simulink model "FanCtl_Spd"  (R2016b)
settings: configuration reference "CodeGenConfigSet" (kept outside this file)
values from neighbouring files (symbols this model uses):
  Fan_numFans_C = Calibration.Parameter    [init_FanCtl_Spd.m]    (also in init_FanCtl_Spd_SIL.m = Simulink.Parameter)
  Fan_rHys2Hi_C = Calibration.Parameter    [init_FanCtl_Spd.m]    (also in init_FanCtl_Spd_SIL.m = Simulink.Parameter)
  Fan_rHys2Lo_C = Calibration.Parameter    [init_FanCtl_Spd.m]    (also in init_FanCtl_Spd_SIL.m = Simulink.Parameter)
  Fan_rHysHi_C = Calibration.Parameter    [init_FanCtl_Spd.m]    (also in init_FanCtl_Spd_SIL.m = Simulink.Parameter)
  Fan_rHysLo_C = Calibration.Parameter    [init_FanCtl_Spd.m]    (also in init_FanCtl_Spd_SIL.m = Simulink.Parameter)
  FanCtl_facCorErr_C = Calibration.Parameter    [init_FanCtl_Spd.m]    (also in init_FanCtl_Spd_SIL.m = Simulink.Parameter)
  FanCtl_facCorSpd2_MAP = Calibration.Parameter    [init_FanCtl_Spd.m]    (also in init_FanCtl_Spd_SIL.m = Simulink.Parameter)
  FanCtl_facCorSpd2_MAPX = Calibration.Parameter    [init_FanCtl_Spd.m]    (also in init_FanCtl_Spd_SIL.m = Simulink.Parameter)
  FanCtl_facCorSpd2_MAPY = Calibration.Parameter    [init_FanCtl_Spd.m]    (also in init_FanCtl_Spd_SIL.m = Simulink.Parameter)
  FanCtl_facCorSpd_MAP = Calibration.Parameter    [init_FanCtl_Spd.m]    (also in init_FanCtl_Spd_SIL.m = Simulink.Parameter)
  FanCtl_facCorSpd_MAPX = Calibration.Parameter    [init_FanCtl_Spd.m]    (also in init_FanCtl_Spd_SIL.m = Simulink.Parameter)
  FanCtl_facCorSpd_MAPY = Calibration.Parameter    [init_FanCtl_Spd.m]    (also in init_FanCtl_Spd_SIL.m = Simulink.Parameter)
  FanCtl_nSpd2Win1L_C = Calibration.Parameter    [init_FanCtl_Spd.m]    (also in init_FanCtl_Spd_SIL.m = Simulink.Parameter)
  FanCtl_nSpd2Win1R_C = Calibration.Parameter    [init_FanCtl_Spd.m]    (also in init_FanCtl_Spd_SIL.m = Simulink.Parameter)
  FanCtl_nSpd2Win2L_C = Calibration.Parameter    [init_FanCtl_Spd.m]    (also in init_FanCtl_Spd_SIL.m = Simulink.Parameter)
  FanCtl_nSpd2Win2R_C = Calibration.Parameter    [init_FanCtl_Spd.m]    (also in init_FanCtl_Spd_SIL.m = Simulink.Parameter)
  FanCtl_nSpd2Win3L_C = Calibration.Parameter    [init_FanCtl_Spd.m]    (also in init_FanCtl_Spd_SIL.m = Simulink.Parameter)
  FanCtl_nSpd2Win3R_C = Calibration.Parameter    [init_FanCtl_Spd.m]    (also in init_FanCtl_Spd_SIL.m = Simulink.Parameter)
  FanCtl_nSpdDes2_MAP = Calibration.Parameter    [init_FanCtl_Spd.m]    (also in init_FanCtl_Spd_SIL.m = Simulink.Parameter)
  FanCtl_nSpdDes2_MAPX = Calibration.Parameter    [init_FanCtl_Spd.m]    (also in init_FanCtl_Spd_SIL.m = Simulink.Parameter)
  FanCtl_nSpdDes2_MAPY = Calibration.Parameter    [init_FanCtl_Spd.m]    (also in init_FanCtl_Spd_SIL.m = Simulink.Parameter)
  FanCtl_nSpdDes_MAP = Calibration.Parameter    [init_FanCtl_Spd.m]    (also in init_FanCtl_Spd_SIL.m = Simulink.Parameter)
  FanCtl_nSpdDes_MAPX = Calibration.Parameter    [init_FanCtl_Spd.m]    (also in init_FanCtl_Spd_SIL.m = Simulink.Parameter)
  FanCtl_nSpdDes_MAPY = Calibration.Parameter    [init_FanCtl_Spd.m]    (also in init_FanCtl_Spd_SIL.m = Simulink.Parameter)
  FanCtl_nSpdFan2Max_C = Calibration.Parameter    [init_FanCtl_Spd.m]    (also in init_FanCtl_Spd_SIL.m = Simulink.Parameter)
  FanCtl_nSpdFanMax_C = Calibration.Parameter    [init_FanCtl_Spd.m]    (also in init_FanCtl_Spd_SIL.m = Simulink.Parameter)
  FanCtl_nSpdMin2_C = Calibration.Parameter    [init_FanCtl_Spd.m]    (also in init_FanCtl_Spd_SIL.m = Simulink.Parameter)
  FanCtl_nSpdMin_C = Calibration.Parameter    [init_FanCtl_Spd.m]    (also in init_FanCtl_Spd_SIL.m = Simulink.Parameter)
  FanCtl_nSpdMinDelta2_C = Calibration.Parameter    [init_FanCtl_Spd.m]    (also in init_FanCtl_Spd_SIL.m = Simulink.Parameter)
  FanCtl_nSpdMinDelta_C = Calibration.Parameter    [init_FanCtl_Spd.m]    (also in init_FanCtl_Spd_SIL.m = Simulink.Parameter)
  FanCtl_nSpdWin1L_C = Calibration.Parameter    [init_FanCtl_Spd.m]    (also in init_FanCtl_Spd_SIL.m = Simulink.Parameter)
  FanCtl_nSpdWin1R_C = Calibration.Parameter    [init_FanCtl_Spd.m]    (also in init_FanCtl_Spd_SIL.m = Simulink.Parameter)
  FanCtl_nSpdWin2L_C = Calibration.Parameter    [init_FanCtl_Spd.m]    (also in init_FanCtl_Spd_SIL.m = Simulink.Parameter)
  FanCtl_nSpdWin2R_C = Calibration.Parameter    [init_FanCtl_Spd.m]    (also in init_FanCtl_Spd_SIL.m = Simulink.Parameter)
  FanCtl_nSpdWin3L_C = Calibration.Parameter    [init_FanCtl_Spd.m]    (also in init_FanCtl_Spd_SIL.m = Simulink.Parameter)
  FanCtl_nSpdWin3R_C = Calibration.Parameter    [init_FanCtl_Spd.m]    (also in init_FanCtl_Spd_SIL.m = Simulink.Parameter)
  FanCtl_rClgDesARMin_C = Calibration.Parameter    [init_FanCtl_Spd.m]    (also in init_FanCtl_Spd_SIL.m = Simulink.Parameter)
  FanCtl_rClgDesErr_C = Calibration.Parameter    [init_FanCtl_Spd.m]    (also in init_FanCtl_Spd_SIL.m = Simulink.Parameter)
  FANCTL_STOFF = fi(1,State_uint8)    [init_FanCtl_Spd.m]    (also in init_FanCtl_Spd_SIL.m)
  FanCtl_tiAftRunMax_C = Calibration.Parameter    [init_FanCtl_Spd.m]    (also in init_FanCtl_Spd_SIL.m = Simulink.Parameter)
  FanCtl_tiDelStrt_C = Calibration.Parameter    [init_FanCtl_Spd.m]    (also in init_FanCtl_Spd_SIL.m = Simulink.Parameter)
  FanCtl_tiTrqResv2_C = Calibration.Parameter    [init_FanCtl_Spd.m]    (also in init_FanCtl_Spd_SIL.m = Simulink.Parameter)
  FanCtl_tiTrqResv_C = Calibration.Parameter    [init_FanCtl_Spd.m]    (also in init_FanCtl_Spd_SIL.m = Simulink.Parameter)
  PRC_100 = fi(100,Prc_100_rate)    [init_FanCtl_Spd.m]    (also in init_FanCtl_Spd_SIL.m)
  PRC_ZERO = fi(0,Prc_100_rate)    [init_FanCtl_Spd.m]    (also in init_FanCtl_Spd_SIL.m)
  STSP_SY = fi(0,State_uint8)    [init_FanCtl_Spd.m]    (also in init_FanCtl_Spd_SIL.m)
undefined symbols (not defined in the file or in its folder): EngState_conv, FanCtl_Spd_DT
libraries: CXLib x12
settings Model: Creator=xinchangran  LastModifiedBy=xinchangran
settings ConfigSetRef: SourceLocation=Base Workspace

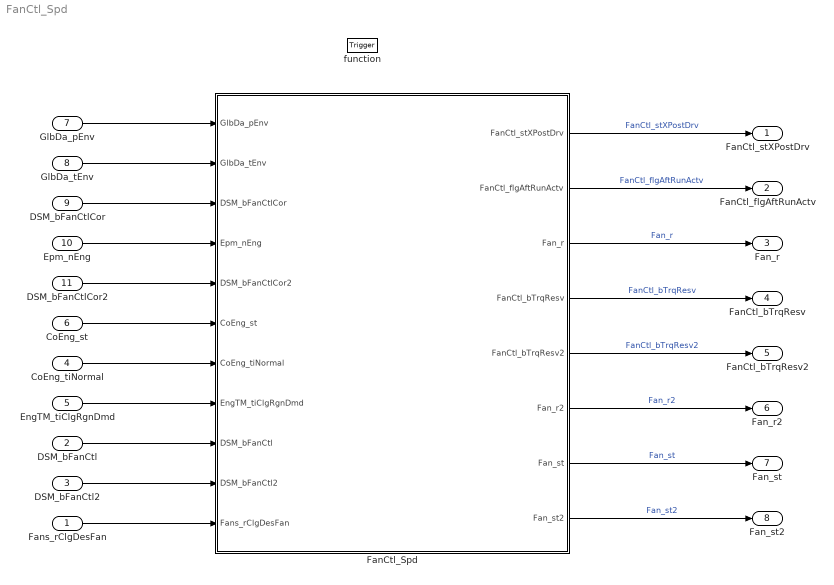
== system FanCtl_Spd ==
  Fans_rClgDesFan : Inport  Tag=%  Description=Relative cooling performance demand to fan  OutMin=-300  OutMax=300  OutDataTypeStr=Prc_100_rate
  DSM_bFanCtl : Inport  Port=2  OutMin=0  OutMax=1  OutDataTypeStr=Dsm
  DSM_bFanCtl2 : Inport  Port=3  OutMin=0  OutMax=1  OutDataTypeStr=Dsm
  CoEng_tiNormal : Inport  Tag=ms  Description="Time since state\"CONENG_RUNNING\"was reached"  Port=4  OutMin=0  OutMax=42949672950  OutDataTypeStr=EngTime_ms
  EngTM_tiClgRgnDmd : Inport  Tag=ms  Description=Duration to keep fan On to cool the DPF and surrounding  Port=5  OutMin=0  OutMax=42949672950  OutDataTypeStr=EngTime_ms
  CoEng_st : Inport  Description=Engine coordinator state  Port=6  OutDataTypeStr=Enum: EngState_conv
  GlbDa_pEnv : Inport  Tag=kPa  Description=environmental pressure  Port=7  OutMin=-3000  OutMax=3000  OutDataTypeStr=AirPressure_kPa
  GlbDa_tEnv : Inport  Tag=deg  Description=environment temperature  Port=8  OutMin=-50  OutMax=150  OutDataTypeStr=Temp_deg
  DSM_bFanCtlCor : Inport  Port=9  OutMin=0  OutMax=1  OutDataTypeStr=Dsm
  Epm_nEng : Inport  Tag=rpm  Description=Engine speed  Port=10  OutMin=0  OutMax=6000  OutDataTypeStr=EngSpeed_rpm
  DSM_bFanCtlCor2 : Inport  Port=11  OutMin=0  OutMax=1  OutDataTypeStr=Dsm
  function : TriggerPort  TriggerType=function-call  VariantControl=Variant
  FanCtl_Spd : Subsystem
  FanCtl_stXPostDrv : Outport  Description=Prolonging post drive due to fan  OutMin=0  OutMax=1  OutDataTypeStr=boolean
  FanCtl_flgAftRunActv : Outport  Description=fan afterrun active  Port=2  OutMin=0  OutMax=1  OutDataTypeStr=boolean
  Fan_r : Outport  Tag=%  Description=Actuator setpoint value for the first fan output  Port=3  OutMin=0  OutMax=100  OutDataTypeStr=DutyCycle_rate
  FanCtl_bTrqResv : Outport  Description=the additional torque required for Fan1 from the engine  Port=4  OutMin=0  OutMax=1  OutDataTypeStr=boolean
  FanCtl_bTrqResv2 : Outport  Description=the additional torque required for Fan2 from the engine  Port=5  OutMin=0  OutMax=1  OutDataTypeStr=boolean
  Fan_r2 : Outport  Tag=%  Description=set point duty cycle for PWM fan power stage 2  Port=6  OutMin=0  OutMax=100  OutDataTypeStr=DutyCycle_rate
  Fan_st : Outport  Description=Fan status based on fan opening  Port=7  OutMin=0  OutMax=1  OutDataTypeStr=boolean
  Fan_st2 : Outport  Description=Fan 2 status based on fan opening  Port=8  OutMin=0  OutMax=1  OutDataTypeStr=boolean
  wires:
  FanCtl_Spd/1(FanCtl_stXPostDrv) -> FanCtl_stXPostDrv/1  "FanCtl_stXPostDrv"
  FanCtl_Spd/2(FanCtl_flgAftRunActv) -> FanCtl_flgAftRunActv/1  "FanCtl_flgAftRunActv"
  FanCtl_Spd/3(Fan_r) -> Fan_r/1  "Fan_r"
  FanCtl_Spd/4(FanCtl_bTrqResv) -> FanCtl_bTrqResv/1  "FanCtl_bTrqResv"
  FanCtl_Spd/5(FanCtl_bTrqResv2) -> FanCtl_bTrqResv2/1  "FanCtl_bTrqResv2"
  FanCtl_Spd/6(Fan_r2) -> Fan_r2/1  "Fan_r2"
  Epm_nEng/1 -> FanCtl_Spd/4(Epm_nEng)
  DSM_bFanCtl2/1 -> FanCtl_Spd/10(DSM_bFanCtl2)
  EngTM_tiClgRgnDmd/1 -> FanCtl_Spd/8(EngTM_tiClgRgnDmd)
  Fans_rClgDesFan/1 -> FanCtl_Spd/11(Fans_rClgDesFan)
  GlbDa_tEnv/1 -> FanCtl_Spd/2(GlbDa_tEnv)
  GlbDa_pEnv/1 -> FanCtl_Spd/1(GlbDa_pEnv)
  DSM_bFanCtlCor2/1 -> FanCtl_Spd/5(DSM_bFanCtlCor2)
  DSM_bFanCtl/1 -> FanCtl_Spd/9(DSM_bFanCtl)
  CoEng_st/1 -> FanCtl_Spd/6(CoEng_st)
  DSM_bFanCtlCor/1 -> FanCtl_Spd/3(DSM_bFanCtlCor)
  CoEng_tiNormal/1 -> FanCtl_Spd/7(CoEng_tiNormal)
  FanCtl_Spd/7(Fan_st) -> Fan_st/1  "Fan_st"
  FanCtl_Spd/8(Fan_st2) -> Fan_st2/1  "Fan_st2"

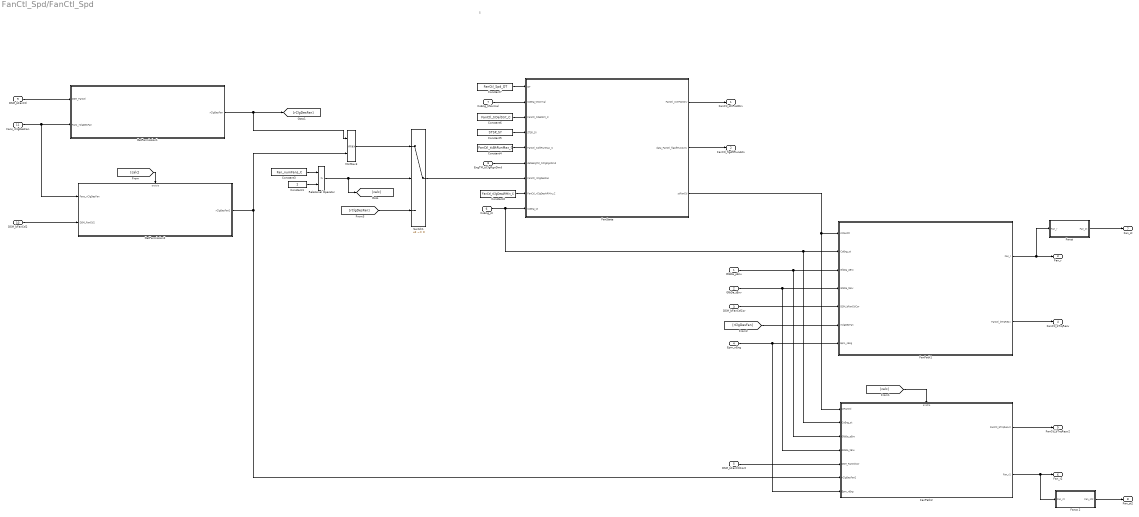
== system FanCtl_Spd/FanCtl_Spd ==
  note: 5
  GlbDa_pEnv : Inport  Tag=%
  GlbDa_tEnv : Inport  Tag=%  Port=2
  DSM_bFanCtlCor : Inport  Tag=%  Port=3
  Epm_nEng : Inport  Tag=%  Port=4
  DSM_bFanCtlCor2 : Inport  Tag=%  Port=5
  CoEng_st : Inport  Port=6
  CoEng_tiNormal : Inport  Port=7
  EngTM_tiClgRgnDmd : Inport  Port=8
  DSM_bFanCtl : Inport  Port=9
  DSM_bFanCtl2 : Inport  Port=10
  Fans_rClgDesFan : Inport  Port=11
  Constant1 : Constant  OutDataTypeStr=Inherit: Inherit via back propagation
  Constant2 : Constant  Value=FanCtl_rClgDesARMin_C
  Constant3 : Constant  Value=Fan_numFans_C
  Constant4 : Constant  Value=FanCtl_tiAftRunMax_C
  Constant5 : Constant  Value=STSP_SY
  Constant6 : Constant  Value=FanCtl_tiDelStrt_C
  Constant7 : Constant  Value=FanCtl_Spd_DT
  FanPath1 : Subsystem
  FanPath2 : Subsystem
  FanState : Subsystem
  "Fanst " : Subsystem
  Fanst 2 : Subsystem
  GetPermission1 : Subsystem
  GetPermission2 : Subsystem
  MinMax3 : MinMax  Function=max  Inputs=2  InputSameDT=on
  Relational Operator : RelationalOperator  Operator=>  OutDataTypeStr=boolean  RndMeth=Simplest
  Switch1 : Switch  Criteria=u2 ~= 0  SaturateOnIntegerOverflow=on  InputSameDT=on
  FanCtl_stXPostDrv : Outport
  FanCtl_flgAftRunActv : Outport  Port=2
  Fan_r : Outport  Tag=%  Port=3  OutMin=0  OutMax=100
  FanCtl_bTrqResv : Outport  Port=4
  FanCtl_bTrqResv2 : Outport  Port=5
  Fan_r2 : Outport  Port=6
  Fan_st : Outport  Tag=%  Port=7
  Fan_st2 : Outport  Tag=%  Port=8
  wires:
  Fans_rClgDesFan/1 -> GetPermission2/1(Fans_rClgDesFan), GetPermission1/2(Fans_rClgDesFan)
  Constant7/1 -> FanState/1(DT)
  Relational Operator/1 -> [calc], Switch1/2
  DSM_bFanCtl/1 -> GetPermission1/1(DSM_FanCtl)
  DSM_bFanCtl2/1 -> GetPermission2/2(DSM_FanCtl2)
  [calc] -> FanPath2/Enable
  Constant6/1 -> FanState/3(FanCtl_tiDelStrt_C)
  Constant5/1 -> FanState/4(STSP_SY)
  [rClgDesFan] -> FanPath1/6(rClgDesFan)
  Switch1/1 -> FanState/7(FanCtl_rClgDesFan)
  FanState/3(stFanCtl) -> FanPath2/1(stFanCtl), FanPath1/1(stFanCtl)
  Constant3/1 -> Relational Operator/1
  GetPermission1/1(rClgDesFan) -> MinMax3/1, [rClgDesFan]
  DSM_bFanCtlCor/1 -> FanPath1/5(DSM_bFanCtlCor)
  Epm_nEng/1 -> FanPath2/7(Epm_nEng), FanPath1/7(Epm_nEng)
  Constant4/1 -> FanState/5(FanCtl_tiAftRunMax_C)
  EngTM_tiClgRgnDmd/1 -> FanState/6(dataEngTM_tiClgRgnDmd)
  FanState/1(FanCtl_stXPostDrv) -> FanCtl_stXPostDrv/1
  GlbDa_tEnv/1 -> FanPath2/4(GlbDa_tEnv), FanPath1/4(GlbDa_tEnv)
  CoEng_tiNormal/1 -> FanState/2(CoEng_tiNormal)
  Constant1/1 -> Relational Operator/2
  MinMax3/1 -> Switch1/1
  FanState/2(data_FanCtl_flgAftRunActv) -> FanCtl_flgAftRunActv/1
  GlbDa_pEnv/1 -> FanPath2/3(GlbDa_pEnv), FanPath1/3(GlbDa_pEnv)
  Constant2/1 -> FanState/8(FanCtl_rClgDesARMin_C)
  FanPath2/1(FanCtl_bTrqResv2) -> FanCtl_bTrqResv2/1
  [calc] -> GetPermission2/Enable
  FanPath2/2(Fan_r2) -> Fanst 2/1(Fan_r2), Fan_r2/1
  FanPath1/2(FanCtl_bTrqResv) -> FanCtl_bTrqResv/1
  FanPath1/1(Fan_r) -> "Fanst "/1(Fan_r), Fan_r/1
  "Fanst "/1(Fan_st) -> Fan_st/1
  GetPermission2/1(rClgDesFan2) -> FanPath2/6(rClgDesFan2), MinMax3/2
  CoEng_st/1 -> FanPath1/2(CoEng_st), FanPath2/2(CoEng_st), FanState/9(CoEng_st)
  DSM_bFanCtlCor2/1 -> FanPath2/5(DSM_FanCtlCor)
  [rClgDesFan] -> Switch1/3
  Fanst 2/1(Fan_st2) -> Fan_st2/1

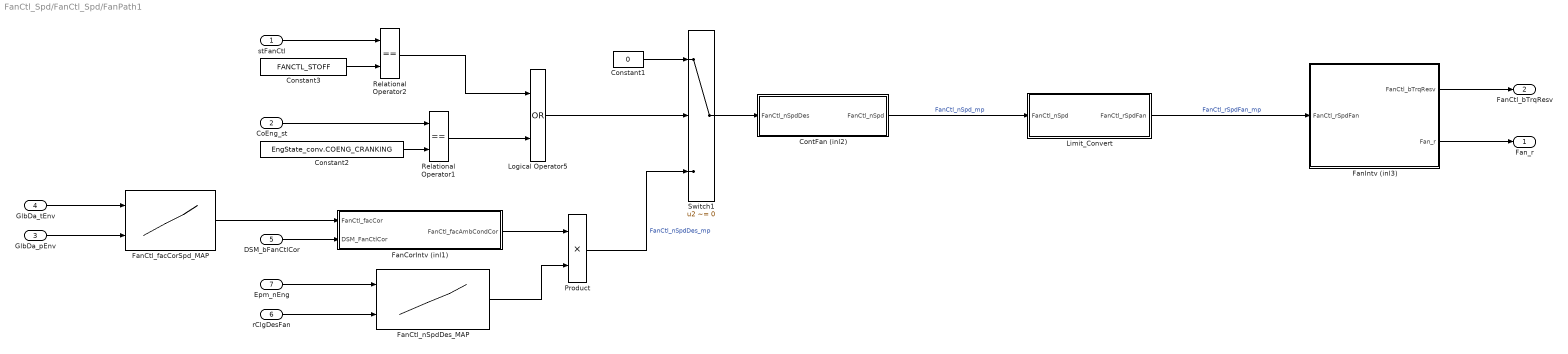
== system FanCtl_Spd/FanCtl_Spd/FanPath1 ==
  stFanCtl : Inport  Tag=%
  CoEng_st : Inport  Tag=%  Port=2
  GlbDa_pEnv : Inport  Tag=%  Port=3
  GlbDa_tEnv : Inport  Tag=%  Port=4
  DSM_bFanCtlCor : Inport  Tag=%  Port=5
  rClgDesFan : Inport  Tag=%  Port=6
  Epm_nEng : Inport  Tag=%  Port=7
  Constant1 : Constant  Value=0  OutDataTypeStr=Inherit: Inherit via back propagation
  Constant2 : Constant  Value=EngState_conv.COENG_CRANKING
  Constant3 : Constant  Value=FANCTL_STOFF
  ContFan (inl2) : Subsystem
  FanCorIntv (inl1) : Subsystem
  FanCtl_facCorSpd_MAP : Lookup_n-D  BreakpointsForDimension1=FanCtl_facCorSpd_MAPY  BreakpointsForDimension2=FanCtl_facCorSpd_MAPX  IndexSearchMethod=Linear search  BeginIndexSearchUsingPreviousIndexResult=on  Table=FanCtl_facCorSpd_MAP  ExtrapMethod=Clip  UseLastTableValue=on  InternalRulePriority=Speed  OutDataTypeStr=Inherit: Inherit via back propagation  SaturateOnIntegerOverflow=on
  FanCtl_nSpdDes_MAP : Lookup_n-D  BreakpointsForDimension1=FanCtl_nSpdDes_MAPY  BreakpointsForDimension2=FanCtl_nSpdDes_MAPX  IndexSearchMethod=Linear search  BeginIndexSearchUsingPreviousIndexResult=on  Table=FanCtl_nSpdDes_MAP  ExtrapMethod=Clip  UseLastTableValue=on  InternalRulePriority=Speed  OutDataTypeStr=Inherit: Inherit via back propagation  SaturateOnIntegerOverflow=on
  FanIntv (inl3) : Subsystem
  Limit_Convert : Subsystem
  Logical Operator5 : Logic  Operator=OR  AllPortsSameDT=off  OutDataTypeStr=boolean
  Product : Product  OutDataTypeStr=Inherit: Inherit via back propagation  SaturateOnIntegerOverflow=on
  Relational Operator1 : RelationalOperator  Operator===  OutDataTypeStr=boolean  RndMeth=Simplest
  Relational Operator2 : RelationalOperator  Operator===  OutDataTypeStr=boolean  RndMeth=Simplest
  Switch1 : Switch  Criteria=u2 ~= 0  SaturateOnIntegerOverflow=on  InputSameDT=on
  Fan_r : Outport  Tag=%
  FanCtl_bTrqResv : Outport  Port=2
  wires:
  FanIntv (inl3)/1(FanCtl_bTrqResv) -> FanCtl_bTrqResv/1
  DSM_bFanCtlCor/1 -> FanCorIntv (inl1)/2(DSM_FanCtlCor)
  FanCtl_facCorSpd_MAP/1 -> FanCorIntv (inl1)/1(FanCtl_facCor)
  Switch1/1 -> ContFan (inl2)/1(FanCtl_nSpdDes)
  Constant1/1 -> Switch1/1
  Limit_Convert/1(FanCtl_rSpdFan) -> FanIntv (inl3)/1(FanCtl_rSpdFan)  "FanCtl_rSpdFan_mp"
  FanCorIntv (inl1)/1(FanCtl_facAmbCondCor) -> Product/1
  FanCtl_nSpdDes_MAP/1 -> Product/2
  FanIntv (inl3)/2(Fan_r) -> Fan_r/1
  ContFan (inl2)/1(FanCtl_nSpd) -> Limit_Convert/1(FanCtl_nSpd)  "FanCtl_nSpd_mp"
  CoEng_st/1 -> Relational Operator1/1
  Relational Operator1/1 -> Logical Operator5/2
  Constant2/1 -> Relational Operator1/2
  Logical Operator5/1 -> Switch1/2
  stFanCtl/1 -> Relational Operator2/1
  Product/1 -> Switch1/3  "FanCtl_nSpdDes_mp"
  Relational Operator2/1 -> Logical Operator5/1
  Constant3/1 -> Relational Operator2/2
  Epm_nEng/1 -> FanCtl_nSpdDes_MAP/1
  rClgDesFan/1 -> FanCtl_nSpdDes_MAP/2
  GlbDa_pEnv/1 -> FanCtl_facCorSpd_MAP/2
  GlbDa_tEnv/1 -> FanCtl_facCorSpd_MAP/1

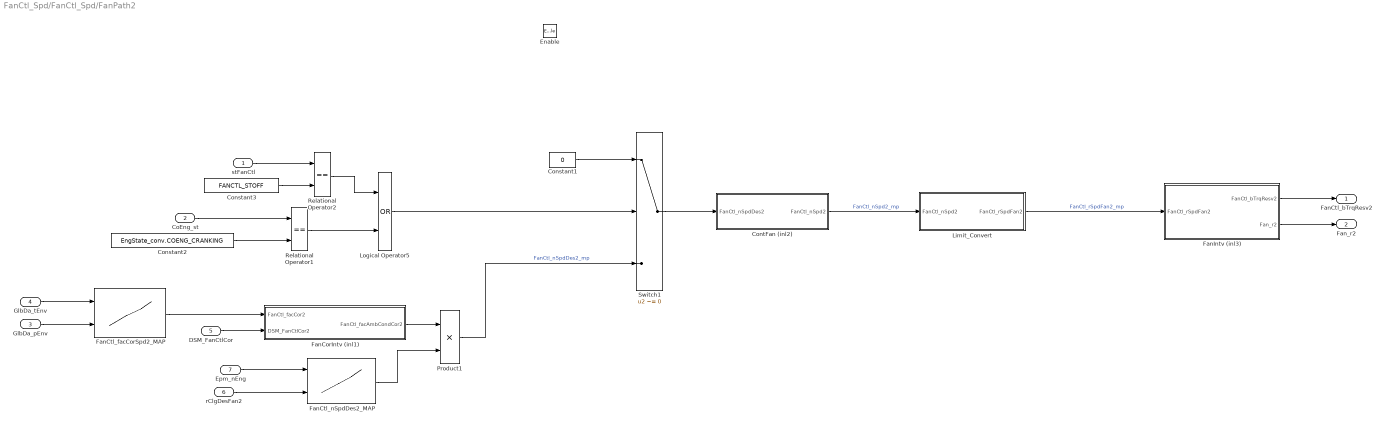
== system FanCtl_Spd/FanCtl_Spd/FanPath2 ==
  stFanCtl : Inport  Tag=%
  CoEng_st : Inport  Tag=%  Port=2
  GlbDa_pEnv : Inport  Tag=%  Port=3
  GlbDa_tEnv : Inport  Tag=%  Port=4
  DSM_FanCtlCor : Inport  Tag=%  Port=5
  rClgDesFan2 : Inport  Tag=%  Port=6
  Epm_nEng : Inport  Tag=%  Port=7
  Enable : EnablePort
  Constant1 : Constant  Value=0  OutDataTypeStr=Inherit: Inherit via back propagation
  Constant2 : Constant  Value=EngState_conv.COENG_CRANKING
  Constant3 : Constant  Value=FANCTL_STOFF
  ContFan (inl2) : Subsystem
  FanCorIntv (inl1) : Subsystem
  FanCtl_facCorSpd2_MAP : Lookup_n-D  BreakpointsForDimension1=FanCtl_facCorSpd2_MAPY  BreakpointsForDimension2=FanCtl_facCorSpd2_MAPX  IndexSearchMethod=Linear search  BeginIndexSearchUsingPreviousIndexResult=on  Table=FanCtl_facCorSpd2_MAP  ExtrapMethod=Clip  UseLastTableValue=on  InternalRulePriority=Speed  OutDataTypeStr=Inherit: Inherit via back propagation  SaturateOnIntegerOverflow=on
  FanCtl_nSpdDes2_MAP : Lookup_n-D  BreakpointsForDimension1=FanCtl_nSpdDes2_MAPY  BreakpointsForDimension2=FanCtl_nSpdDes2_MAPX  IndexSearchMethod=Linear search  BeginIndexSearchUsingPreviousIndexResult=on  Table=FanCtl_nSpdDes2_MAP  ExtrapMethod=Clip  UseLastTableValue=on  InternalRulePriority=Speed  OutDataTypeStr=Inherit: Inherit via back propagation  SaturateOnIntegerOverflow=on
  FanIntv (inl3) : Subsystem
  Limit_Convert : Subsystem
  Logical Operator5 : Logic  Operator=OR  AllPortsSameDT=off  OutDataTypeStr=boolean
  Product1 : Product  OutDataTypeStr=Inherit: Inherit via back propagation  SaturateOnIntegerOverflow=on
  Relational Operator1 : RelationalOperator  Operator===  OutDataTypeStr=boolean  RndMeth=Simplest
  Relational Operator2 : RelationalOperator  Operator===  OutDataTypeStr=boolean  RndMeth=Simplest
  Switch1 : Switch  Criteria=u2 ~= 0  SaturateOnIntegerOverflow=on  InputSameDT=on
  FanCtl_bTrqResv2 : Outport
  Fan_r2 : Outport  Port=2
  wires:
  Product1/1 -> Switch1/3  "FanCtl_nSpdDes2_mp"
  Relational Operator2/1 -> Logical Operator5/1
  Logical Operator5/1 -> Switch1/2
  Constant2/1 -> Relational Operator1/2
  Constant3/1 -> Relational Operator2/2
  Relational Operator1/1 -> Logical Operator5/2
  CoEng_st/1 -> Relational Operator1/1
  ContFan (inl2)/1(FanCtl_nSpd2) -> Limit_Convert/1(FanCtl_nSpd2)  "FanCtl_nSpd2_mp"
  FanIntv (inl3)/2(Fan_r2) -> Fan_r2/1
  FanCtl_nSpdDes2_MAP/1 -> Product1/2
  FanCorIntv (inl1)/1(FanCtl_facAmbCondCor2) -> Product1/1
  Limit_Convert/1(FanCtl_rSpdFan2) -> FanIntv (inl3)/1(FanCtl_rSpdFan2)  "FanCtl_rSpdFan2_mp"
  Constant1/1 -> Switch1/1
  Switch1/1 -> ContFan (inl2)/1(FanCtl_nSpdDes2)
  FanCtl_facCorSpd2_MAP/1 -> FanCorIntv (inl1)/1(FanCtl_facCor2)
  stFanCtl/1 -> Relational Operator2/1
  DSM_FanCtlCor/1 -> FanCorIntv (inl1)/2(DSM_FanCtlCor2)
  FanIntv (inl3)/1(FanCtl_bTrqResv2) -> FanCtl_bTrqResv2/1
  GlbDa_pEnv/1 -> FanCtl_facCorSpd2_MAP/2
  GlbDa_tEnv/1 -> FanCtl_facCorSpd2_MAP/1
  rClgDesFan2/1 -> FanCtl_nSpdDes2_MAP/2
  Epm_nEng/1 -> FanCtl_nSpdDes2_MAP/1

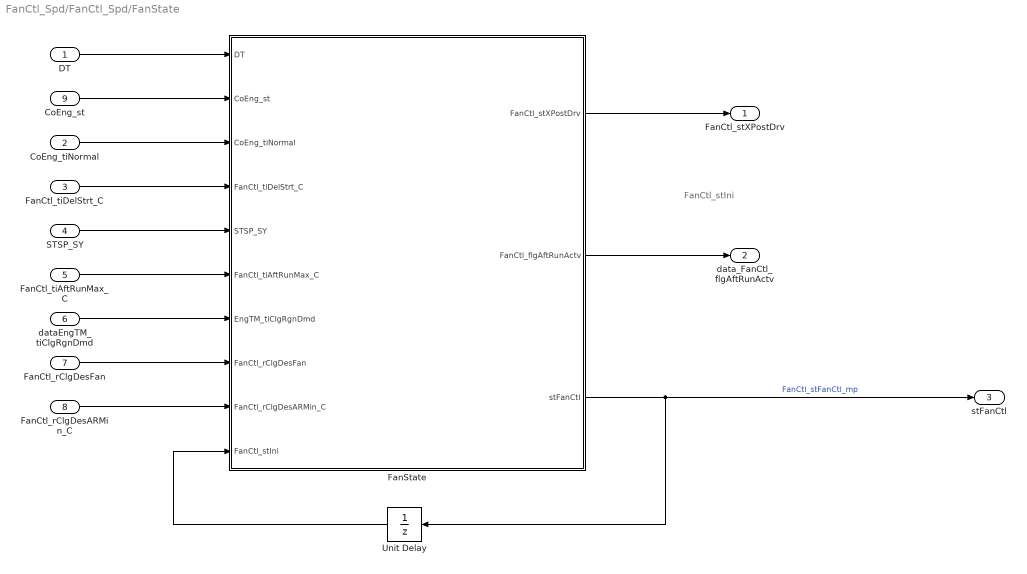
== system FanCtl_Spd/FanCtl_Spd/FanState ==
  note: FanCtl_stIni
  DT : Inport
  CoEng_tiNormal : Inport  Port=2
  FanCtl_tiDelStrt_C : Inport  Port=3
  STSP_SY : Inport  Port=4
  FanCtl_tiAftRunMax_C : Inport  Port=5
  dataEngTM_tiClgRgnDmd : Inport  Port=6
  FanCtl_rClgDesFan : Inport  Port=7
  FanCtl_rClgDesARMin_C : Inport  Port=8
  CoEng_st : Inport  Port=9
  FanState : Stateflow chart  TreatAsAtomicUnit=on
  Unit Delay : UnitDelay  SampleTime=-1
      settings: AttributesFormatString=InitialValue=%<InitialCondition>
  FanCtl_stXPostDrv : Outport
  data_FanCtl_flgAftRunActv : Outport  Port=2
  stFanCtl : Outport  Port=3
  wires:
  FanState/3(stFanCtl) -> stFanCtl/1, Unit Delay/1  "FanCtl_stFanCtl_mp"
  DT/1 -> FanState/1(DT)
  FanCtl_rClgDesARMin_C/1 -> FanState/9(FanCtl_rClgDesARMin_C)
  CoEng_tiNormal/1 -> FanState/3(CoEng_tiNormal)
  FanState/2(FanCtl_flgAftRunActv) -> data_FanCtl_flgAftRunActv/1
  FanCtl_tiDelStrt_C/1 -> FanState/4(FanCtl_tiDelStrt_C)
  CoEng_st/1 -> FanState/2(CoEng_st)
  STSP_SY/1 -> FanState/5(STSP_SY)
  FanCtl_tiAftRunMax_C/1 -> FanState/6(FanCtl_tiAftRunMax_C)
  dataEngTM_tiClgRgnDmd/1 -> FanState/7(EngTM_tiClgRgnDmd)
  FanCtl_rClgDesFan/1 -> FanState/8(FanCtl_rClgDesFan)
  Unit Delay/1 -> FanState/10(FanCtl_stIni)
  FanState/1(FanCtl_stXPostDrv) -> FanCtl_stXPostDrv/1

== system FanCtl_Spd/FanCtl_Spd/Fanst  ==
  Fan_r : Inport
  Constant8 : Constant  Value=Fan_rHysLo_C
  Constant9 : Constant  Value=Fan_rHysHi_C
  Hysteresis_S16 : CXLib/Hysteresis_S16
  Fan_st : Outport
  wires:
  Constant8/1 -> Hysteresis_S16/2
  Constant9/1 -> Hysteresis_S16/3
  Hysteresis_S16/1 -> Fan_st/1
  Fan_r/1 -> Hysteresis_S16/1

== system FanCtl_Spd/FanCtl_Spd/Fanst 2 ==
  Fan_r2 : Inport
  Constant8 : Constant  Value=Fan_rHys2Lo_C
  Constant9 : Constant  Value=Fan_rHys2Hi_C
  Hysteresis_S16 : CXLib/Hysteresis_S16
  Fan_st2 : Outport
  wires:
  Fan_r2/1 -> Hysteresis_S16/1
  Hysteresis_S16/1 -> Fan_st2/1
  Constant9/1 -> Hysteresis_S16/3
  Constant8/1 -> Hysteresis_S16/2

== system FanCtl_Spd/FanCtl_Spd/GetPermission1 ==
  DSM_FanCtl : Inport
  Fans_rClgDesFan : Inport  Port=2
  Constant2 : Constant  Value=FanCtl_rClgDesErr_C
  Switch1 : Switch  Criteria=u2 ~= 0  SaturateOnIntegerOverflow=on  InputSameDT=on
  rClgDesFan : Outport
  wires:
  DSM_FanCtl/1 -> Switch1/2
  Switch1/1 -> rClgDesFan/1
  Fans_rClgDesFan/1 -> Switch1/1
  Constant2/1 -> Switch1/3

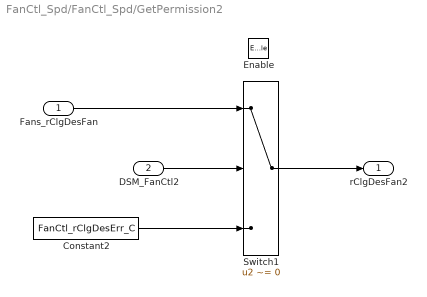
== system FanCtl_Spd/FanCtl_Spd/GetPermission2 ==
  Fans_rClgDesFan : Inport
  DSM_FanCtl2 : Inport  Port=2
  Enable : EnablePort
  Constant2 : Constant  Value=FanCtl_rClgDesErr_C
  Switch1 : Switch  Criteria=u2 ~= 0  SaturateOnIntegerOverflow=on  InputSameDT=on
  rClgDesFan2 : Outport
  wires:
  Switch1/1 -> rClgDesFan2/1
  DSM_FanCtl2/1 -> Switch1/2
  Fans_rClgDesFan/1 -> Switch1/1
  Constant2/1 -> Switch1/3

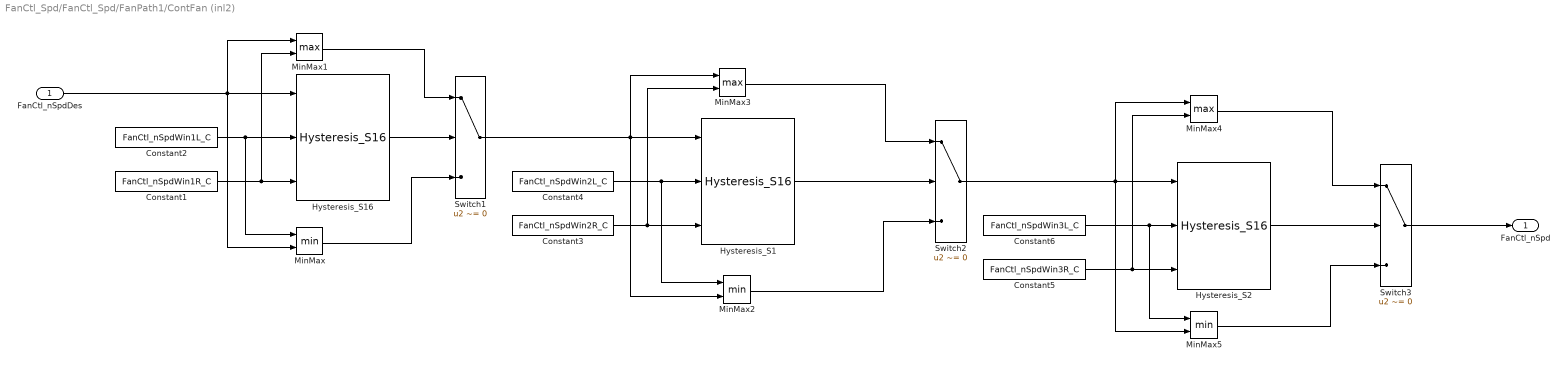
== system FanCtl_Spd/FanCtl_Spd/FanPath1/ContFan (inl2) ==
  FanCtl_nSpdDes : Inport  Tag=%
  Constant1 : Constant  Value=FanCtl_nSpdWin1R_C
  Constant2 : Constant  Value=FanCtl_nSpdWin1L_C
  Constant3 : Constant  Value=FanCtl_nSpdWin2R_C
  Constant4 : Constant  Value=FanCtl_nSpdWin2L_C
  Constant5 : Constant  Value=FanCtl_nSpdWin3R_C
  Constant6 : Constant  Value=FanCtl_nSpdWin3L_C
  Hysteresis_S1 : CXLib/Hysteresis_S16
  Hysteresis_S16 : CXLib/Hysteresis_S16
  Hysteresis_S2 : CXLib/Hysteresis_S16
  MinMax : MinMax  Inputs=2
  MinMax1 : MinMax  Function=max  Inputs=2
  MinMax2 : MinMax  Inputs=2
  MinMax3 : MinMax  Function=max  Inputs=2
  MinMax4 : MinMax  Function=max  Inputs=2
  MinMax5 : MinMax  Inputs=2
  Switch1 : Switch  Criteria=u2 ~= 0  SaturateOnIntegerOverflow=on  InputSameDT=on
  Switch2 : Switch  Criteria=u2 ~= 0  SaturateOnIntegerOverflow=on  InputSameDT=on
  Switch3 : Switch  Criteria=u2 ~= 0  SaturateOnIntegerOverflow=on  InputSameDT=on
  FanCtl_nSpd : Outport
  wires:
  FanCtl_nSpdDes/1 -> Hysteresis_S16/1, MinMax/2, MinMax1/1
  Hysteresis_S16/1 -> Switch1/2
  Constant1/1 -> Hysteresis_S16/3, MinMax1/2
  Constant2/1 -> Hysteresis_S16/2, MinMax/1
  MinMax/1 -> Switch1/3
  MinMax1/1 -> Switch1/1
  Switch1/1 -> Hysteresis_S1/1, MinMax3/1, MinMax2/2
  Constant4/1 -> Hysteresis_S1/2, MinMax2/1
  Constant3/1 -> Hysteresis_S1/3, MinMax3/2
  Hysteresis_S1/1 -> Switch2/2
  MinMax2/1 -> Switch2/3
  MinMax3/1 -> Switch2/1
  Hysteresis_S2/1 -> Switch3/2
  MinMax4/1 -> Switch3/1
  MinMax5/1 -> Switch3/3
  Switch3/1 -> FanCtl_nSpd/1
  Switch2/1 -> Hysteresis_S2/1, MinMax4/1, MinMax5/2
  Constant6/1 -> Hysteresis_S2/2, MinMax5/1
  Constant5/1 -> Hysteresis_S2/3, MinMax4/2

== system FanCtl_Spd/FanCtl_Spd/FanPath1/FanCorIntv (inl1) ==
  FanCtl_facCor : Inport  Tag=%
  DSM_FanCtlCor : Inport  Tag=%  Port=2
  Constant2 : Constant  Value=FanCtl_facCorErr_C
  Switch1 : Switch  Criteria=u2 ~= 0  SaturateOnIntegerOverflow=on  InputSameDT=on
  FanCtl_facAmbCondCor : Outport
  wires:
  Constant2/1 -> Switch1/3
  FanCtl_facCor/1 -> Switch1/1
  Switch1/1 -> FanCtl_facAmbCondCor/1
  DSM_FanCtlCor/1 -> Switch1/2

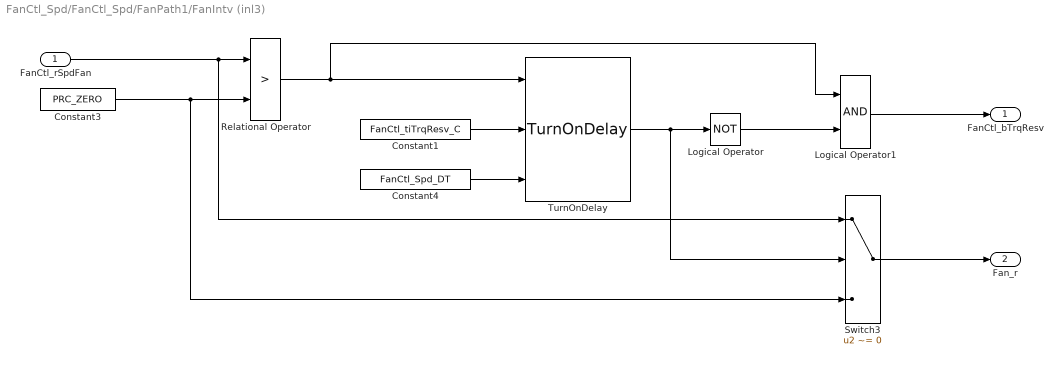
== system FanCtl_Spd/FanCtl_Spd/FanPath1/FanIntv (inl3) ==
  FanCtl_rSpdFan : Inport  Tag=%
  Constant1 : Constant  Value=FanCtl_tiTrqResv_C  SampleTime=-1
  Constant3 : Constant  Value=PRC_ZERO  OutDataTypeStr=Inherit: Inherit via back propagation
  Constant4 : Constant  Value=FanCtl_Spd_DT  SampleTime=-1
  Logical Operator : Logic  Operator=NOT  AllPortsSameDT=off  OutDataTypeStr=boolean
  Logical Operator1 : Logic  AllPortsSameDT=off  OutDataTypeStr=boolean
  Relational Operator : RelationalOperator  Operator=>  OutDataTypeStr=boolean  RndMeth=Simplest
  Switch3 : Switch  Criteria=u2 ~= 0  SaturateOnIntegerOverflow=on  InputSameDT=on
  TurnOnDelay : CXLib/TurnOnDelay
  FanCtl_bTrqResv : Outport
  Fan_r : Outport  Port=2
  wires:
  FanCtl_rSpdFan/1 -> Switch3/1, Relational Operator/1
  Constant3/1 -> Relational Operator/2, Switch3/3
  Relational Operator/1 -> TurnOnDelay/1, Logical Operator1/1
  TurnOnDelay/1 -> Logical Operator/1, Switch3/2
  Logical Operator/1 -> Logical Operator1/2
  Logical Operator1/1 -> FanCtl_bTrqResv/1
  Switch3/1 -> Fan_r/1
  Constant4/1 -> TurnOnDelay/3
  Constant1/1 -> TurnOnDelay/2

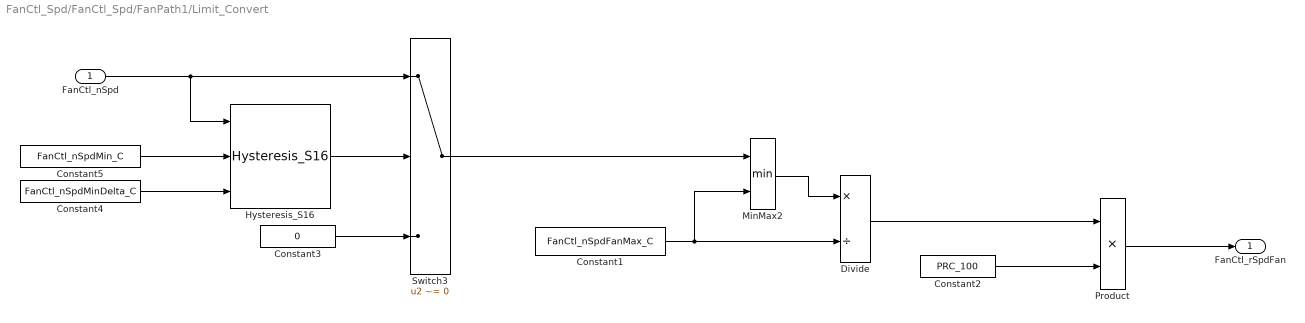
== system FanCtl_Spd/FanCtl_Spd/FanPath1/Limit_Convert ==
  FanCtl_nSpd : Inport  Tag=%
  Constant1 : Constant  Value=FanCtl_nSpdFanMax_C
  Constant2 : Constant  Value=PRC_100  OutDataTypeStr=Inherit: Inherit via back propagation
  Constant3 : Constant  Value=0  OutDataTypeStr=Inherit: Inherit via back propagation
  Constant4 : Constant  Value=FanCtl_nSpdMinDelta_C
  Constant5 : Constant  Value=FanCtl_nSpdMin_C
  Divide : Product  Inputs=*/  OutDataTypeStr=fixdt(1,32,100000^-1,0)  SaturateOnIntegerOverflow=on
  Hysteresis_S16 : CXLib/Hysteresis_S16
  MinMax2 : MinMax  Inputs=2
  Product : Product  OutDataTypeStr=Inherit: Inherit via back propagation  SaturateOnIntegerOverflow=on
  Switch3 : Switch  Criteria=u2 ~= 0  SaturateOnIntegerOverflow=on  InputSameDT=on
  FanCtl_rSpdFan : Outport
  wires:
  Product/1 -> FanCtl_rSpdFan/1
  Constant2/1 -> Product/2
  Constant1/1 -> MinMax2/2, Divide/2
  MinMax2/1 -> Divide/1
  Switch3/1 -> MinMax2/1
  Constant3/1 -> Switch3/3
  FanCtl_nSpd/1 -> Hysteresis_S16/1, Switch3/1
  Hysteresis_S16/1 -> Switch3/2
  Constant5/1 -> Hysteresis_S16/2
  Constant4/1 -> Hysteresis_S16/3
  Divide/1 -> Product/1

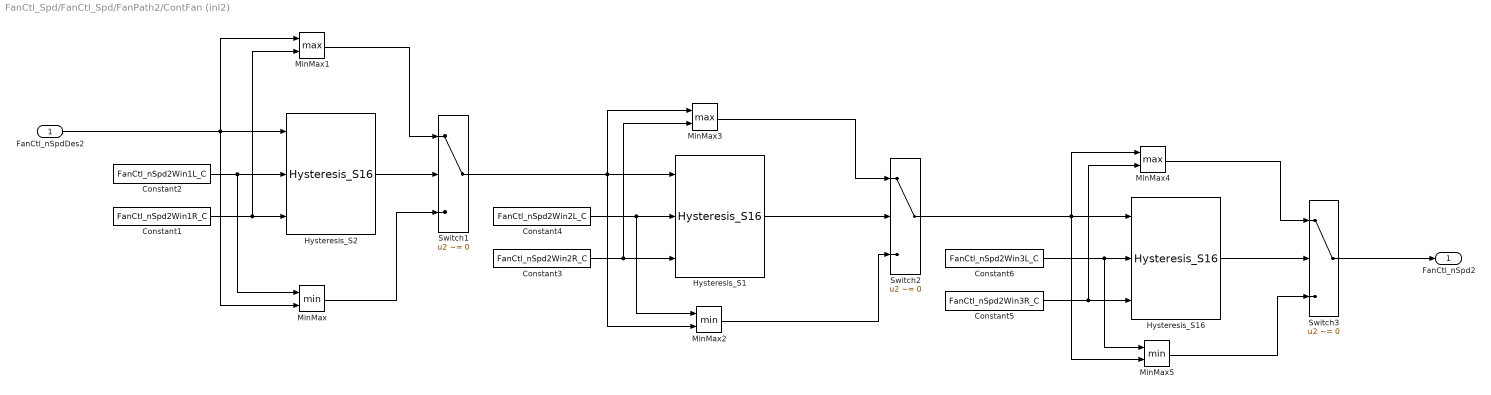
== system FanCtl_Spd/FanCtl_Spd/FanPath2/ContFan (inl2) ==
  FanCtl_nSpdDes2 : Inport  Tag=%
  Constant1 : Constant  Value=FanCtl_nSpd2Win1R_C
  Constant2 : Constant  Value=FanCtl_nSpd2Win1L_C
  Constant3 : Constant  Value=FanCtl_nSpd2Win2R_C
  Constant4 : Constant  Value=FanCtl_nSpd2Win2L_C
  Constant5 : Constant  Value=FanCtl_nSpd2Win3R_C
  Constant6 : Constant  Value=FanCtl_nSpd2Win3L_C
  Hysteresis_S1 : CXLib/Hysteresis_S16
  Hysteresis_S16 : CXLib/Hysteresis_S16
  Hysteresis_S2 : CXLib/Hysteresis_S16
  MinMax : MinMax  Inputs=2
  MinMax1 : MinMax  Function=max  Inputs=2
  MinMax2 : MinMax  Inputs=2
  MinMax3 : MinMax  Function=max  Inputs=2
  MinMax4 : MinMax  Function=max  Inputs=2
  MinMax5 : MinMax  Inputs=2
  Switch1 : Switch  Criteria=u2 ~= 0  SaturateOnIntegerOverflow=on  InputSameDT=on
  Switch2 : Switch  Criteria=u2 ~= 0  SaturateOnIntegerOverflow=on  InputSameDT=on
  Switch3 : Switch  Criteria=u2 ~= 0  SaturateOnIntegerOverflow=on  InputSameDT=on
  FanCtl_nSpd2 : Outport
  wires:
  Constant5/1 -> Hysteresis_S16/3, MinMax4/2
  Constant6/1 -> MinMax5/1, Hysteresis_S16/2
  Switch2/1 -> Hysteresis_S16/1, MinMax5/2, MinMax4/1
  Switch3/1 -> FanCtl_nSpd2/1
  MinMax5/1 -> Switch3/3
  MinMax4/1 -> Switch3/1
  Hysteresis_S16/1 -> Switch3/2
  MinMax3/1 -> Switch2/1
  MinMax2/1 -> Switch2/3
  Hysteresis_S1/1 -> Switch2/2
  Constant3/1 -> Hysteresis_S1/3, MinMax3/2
  Constant4/1 -> Hysteresis_S1/2, MinMax2/1
  Switch1/1 -> Hysteresis_S1/1, MinMax2/2, MinMax3/1
  MinMax1/1 -> Switch1/1
  MinMax/1 -> Switch1/3
  Constant2/1 -> Hysteresis_S2/2, MinMax/1
  Constant1/1 -> Hysteresis_S2/3, MinMax1/2
  Hysteresis_S2/1 -> Switch1/2
  FanCtl_nSpdDes2/1 -> Hysteresis_S2/1, MinMax1/1, MinMax/2

== system FanCtl_Spd/FanCtl_Spd/FanPath2/FanCorIntv (inl1) ==
  FanCtl_facCor2 : Inport  Tag=%
  DSM_FanCtlCor2 : Inport  Tag=%  Port=2
  Constant2 : Constant  Value=FanCtl_facCorErr_C
  Switch1 : Switch  Criteria=u2 ~= 0  SaturateOnIntegerOverflow=on  InputSameDT=on
  FanCtl_facAmbCondCor2 : Outport
  wires:
  DSM_FanCtlCor2/1 -> Switch1/2
  Switch1/1 -> FanCtl_facAmbCondCor2/1
  FanCtl_facCor2/1 -> Switch1/1
  Constant2/1 -> Switch1/3

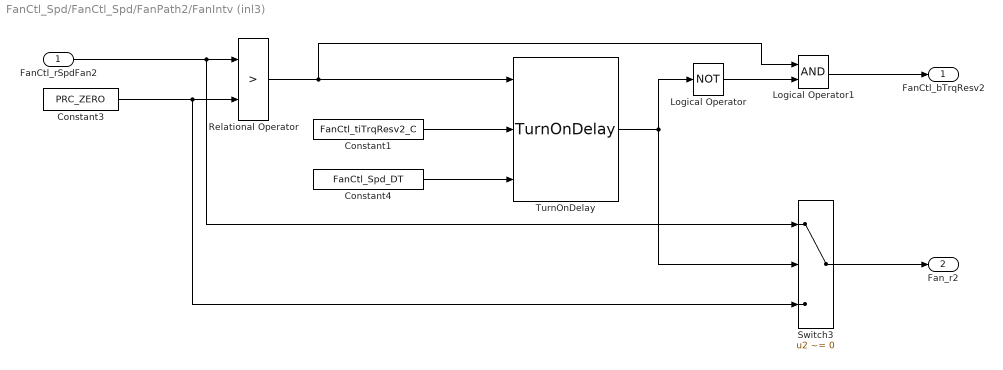
== system FanCtl_Spd/FanCtl_Spd/FanPath2/FanIntv (inl3) ==
  FanCtl_rSpdFan2 : Inport  Tag=%
  Constant1 : Constant  Value=FanCtl_tiTrqResv2_C  SampleTime=-1
  Constant3 : Constant  Value=PRC_ZERO  OutDataTypeStr=Inherit: Inherit via back propagation
  Constant4 : Constant  Value=FanCtl_Spd_DT  SampleTime=-1
  Logical Operator : Logic  Operator=NOT  AllPortsSameDT=off  OutDataTypeStr=boolean
  Logical Operator1 : Logic  AllPortsSameDT=off  OutDataTypeStr=boolean
  Relational Operator : RelationalOperator  Operator=>  OutDataTypeStr=boolean  RndMeth=Simplest
  Switch3 : Switch  Criteria=u2 ~= 0  SaturateOnIntegerOverflow=on  InputSameDT=on
  TurnOnDelay : CXLib/TurnOnDelay
  FanCtl_bTrqResv2 : Outport
  Fan_r2 : Outport  Port=2
  wires:
  Constant1/1 -> TurnOnDelay/2
  Constant4/1 -> TurnOnDelay/3
  Switch3/1 -> Fan_r2/1
  Logical Operator1/1 -> FanCtl_bTrqResv2/1
  Logical Operator/1 -> Logical Operator1/2
  TurnOnDelay/1 -> Switch3/2, Logical Operator/1
  Relational Operator/1 -> TurnOnDelay/1, Logical Operator1/1
  Constant3/1 -> Switch3/3, Relational Operator/2
  FanCtl_rSpdFan2/1 -> Relational Operator/1, Switch3/1

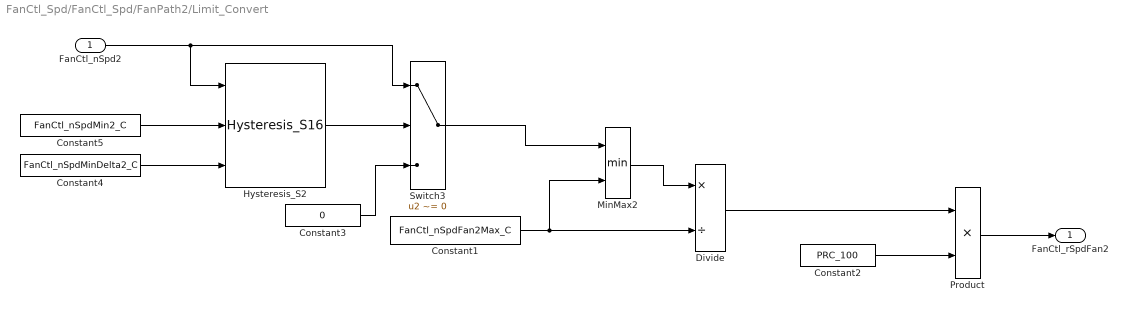
== system FanCtl_Spd/FanCtl_Spd/FanPath2/Limit_Convert ==
  FanCtl_nSpd2 : Inport  Tag=%
  Constant1 : Constant  Value=FanCtl_nSpdFan2Max_C
  Constant2 : Constant  Value=PRC_100  OutDataTypeStr=Inherit: Inherit via back propagation
  Constant3 : Constant  Value=0  OutDataTypeStr=Inherit: Inherit via back propagation
  Constant4 : Constant  Value=FanCtl_nSpdMinDelta2_C
  Constant5 : Constant  Value=FanCtl_nSpdMin2_C
  Divide : Product  Inputs=*/  OutDataTypeStr=fixdt(1,32,100000^-1,0)  SaturateOnIntegerOverflow=on
  Hysteresis_S2 : CXLib/Hysteresis_S16
  MinMax2 : MinMax  Inputs=2
  Product : Product  OutDataTypeStr=Inherit: Inherit via back propagation  SaturateOnIntegerOverflow=on
  Switch3 : Switch  Criteria=u2 ~= 0  SaturateOnIntegerOverflow=on  InputSameDT=on
  FanCtl_rSpdFan2 : Outport
  wires:
  Divide/1 -> Product/1
  Constant4/1 -> Hysteresis_S2/3
  Constant5/1 -> Hysteresis_S2/2
  Hysteresis_S2/1 -> Switch3/2
  FanCtl_nSpd2/1 -> Hysteresis_S2/1, Switch3/1
  Constant3/1 -> Switch3/3
  Switch3/1 -> MinMax2/1
  MinMax2/1 -> Divide/1
  Constant1/1 -> Divide/2, MinMax2/2
  Constant2/1 -> Product/2
  Product/1 -> FanCtl_rSpdFan2/1

== stateflow chart FanCtl_Spd/FanState/FanState ==
  state FanCtl_StNormal
    entry:stFanCtl =2;
    FanCtl_tiSt = 0;
    during:FanCtl_tiSt = FanCtl_tiSt + DT;
  state FanCtl_StOff
    entry:stFanCtl = 1;
    FanCtl_tiSt = 0;
    FanCtl_stXPostDrv = 0;
    FanCtl_flgAftRunActv = 0;
    during:FanCtl_tiSt = FanCtl_tiSt + DT;
  state FanCtl_StAfterRun
    entry:stFanCtl =3;
    FanCtl_stXPostDrv = 1;
    FanCtl_flgAftRunActv = 1;
    during:FanCtl_tiSt = FanCtl_tiSt +DT;
  FanCtl_StNormal -> FanCtl_StAfterRun : %FanCtl_stCalc_Proc%
      | [((STSP_SY > 0)&&(CoEng_st == EngState_conv.COENG_FINISH)|| (CoEng_st == EngState_conv.COENG_READY))||CoEng_st == EngState_conv.COENG_FINISH]
  FanCtl_StOff -> FanCtl_StNormal [order 1] : %FanCtl_stCalc_Proc%
      | [(CoEng_st == EngState_conv.COENG_RUNNING)&&...
      | (CoEng_tiNormal > FanCtl_tiDelStrt_C)]
  (default) -> FanCtl_StOff
  FanCtl_StOff -> FanCtl_StOff [order 2] : [FanCtl_stIni == 1]
  FanCtl_StAfterRun -> FanCtl_StOff [order 1] : %FanCtl_stCalc_Proc%
      | [(FanCtl_tiSt >max( FanCtl_tiAftRunMax_C, EngTM_tiClgRgnDmd))||...
      | (FanCtl_rClgDesFan <= FanCtl_rClgDesARMin_C)||(CoEng_st == EngState_conv.COENG_RUNNING)]
  FanCtl_StAfterRun -> FanCtl_StAfterRun [order 2] : [FanCtl_stIni == 3]
  data: FanCtl_stXPostDrv output; FanCtl_flgAftRunActv output; stFanCtl output uint8; DT input; CoEng_st input; CoEng_tiNormal input; FanCtl_tiDelStrt_C input; STSP_SY input; FanCtl_tiAftRunMax_C input; EngTM_tiClgRgnDmd input; FanCtl_rClgDesFan input; FanCtl_rClgDesARMin_C input; FanCtl_tiSt local uint32; FANCTL_STNORMAL constant uint8; FANCTL_STOFF constant uint8; FANCTL_STAFTRUN constant uint8; FanCtl_stIni input uint8
